simulink model "iter_imas_sc1_Zc_2"  (Simulink 8.5)
settings: Solver=ode1  StartTime=EqTime  StopTime=1e8  FixedStep=SimStep  MaxStep=5.e-3  MinStep=2e-4  RelTol=1.e-3
undefined symbols (not defined in the file): A_currterm, A_div, A_divrd, A_lim, A_vs, A_vs_hl, Acd2, B_currterm, B_div, B_divrd, B_lim, B_vs, B_vs_hl, Bcd2, C_currterm, C_div, C_divrd, C_lim, C_vs, C_vs_hl, Ccd2, D_currterm, D_div, D_divrd, D_lim, D_vs, D_vs_hl, Dcd2, Imax, key_imas, n_gaps, ncam, npf, ntur, RupRd, scr_data, SimStep, Vcspf_up, vec_imas, volt
libraries: simulink x57
(part 1 of 2)
settings Model: Creator=Kavin  ModifiedByFormat=Kavin  LastModifiedBy=Kavin  ExtModeTrigMode=oneshot  ExtModeArmWhenConnect=off  ExtModeAutoUpdateStatusClock=off
settings DataIOCC: LimitDataPoints=off  TimeSaveName=sim_time  SignalLoggingName=sigsOut
settings OptimizationCC: BooleanDataType=off  OptimizeBlockIOStorage=off  BufferReuse=off  GlobalBufferReuse=off  ExpressionFolding=off  ExpressionDepthLimit=128  LocalBlockOutputs=off  InitFltsAndDblsToZero=on
settings DebuggingCC: SaveWithParameterizedLinksMsg=none  SignalResolutionControl=TryResolveAllWithWarning  MultiTaskDSMMsg=warning  MultiTaskCondExecSysMsg=none  FcnCallInpInsideContextMsg=UseLocalSettings  StateNameClashWarn=none
settings HardwareCC: TargetUnknown=on
settings CodeAppCC: IgnoreCustomStorageClasses=off
settings GRTTargetCC: TargetFcnLib=ansi_tfl_tmw.mat

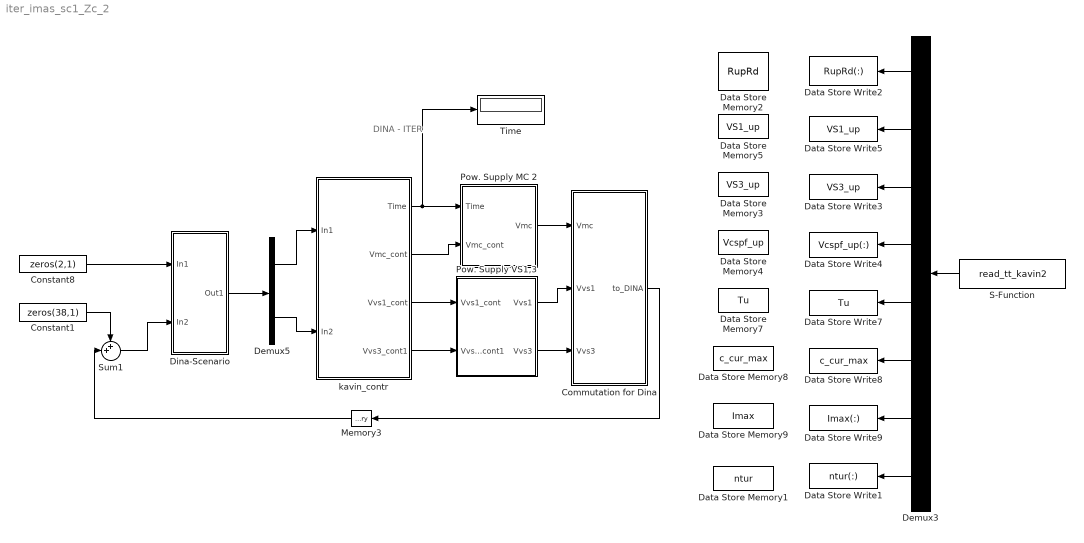
== system iter_imas_sc1_Zc_2 ==
  note: DINA - ITER
  Commutation for Dina : Subsystem
  Constant1 : Constant  Value=zeros(38,1)
  Constant8 : Constant  Value=zeros(2,1)
  Data Store Memory1 : DataStoreMemory  DataStoreName=ntur  ReadBeforeWriteMsg=warning  WriteAfterWriteMsg=warning  WriteAfterReadMsg=warning  InitialValue="[554,554,554,554,554  248.6 115.2 185.9 169.9 216.8  459.4 1]"
  Data Store Memory2 : DataStoreMemory  DataStoreName=RupRd  ReadBeforeWriteMsg=warning  WriteAfterWriteMsg=warning  WriteAfterReadMsg=warning  InitialValue=[1; ones(5,1)*1e-6]
  Data Store Memory3 : DataStoreMemory  DataStoreName=VS3_up  ReadBeforeWriteMsg=warning  WriteAfterWriteMsg=warning  WriteAfterReadMsg=warning
  Data Store Memory4 : DataStoreMemory  DataStoreName=Vcspf_up  ReadBeforeWriteMsg=warning  WriteAfterWriteMsg=warning  WriteAfterReadMsg=warning  InitialValue=zeros(11,1)
  Data Store Memory5 : DataStoreMemory  DataStoreName=VS1_up  ReadBeforeWriteMsg=warning  WriteAfterWriteMsg=warning  WriteAfterReadMsg=warning
  Data Store Memory7 : DataStoreMemory  DataStoreName=Tu  ReadBeforeWriteMsg=warning  WriteAfterWriteMsg=warning  WriteAfterReadMsg=warning
  Data Store Memory8 : DataStoreMemory  DataStoreName=c_cur_max  ReadBeforeWriteMsg=warning  WriteAfterWriteMsg=warning  WriteAfterReadMsg=warning
  Data Store Memory9 : DataStoreMemory  DataStoreName=Imax  ReadBeforeWriteMsg=warning  WriteAfterWriteMsg=warning  WriteAfterReadMsg=warning  InitialValue=ones(1,11)*1e6
  Data Store Write1 : DataStoreWrite  DataStoreName=ntur  DataStoreElements=ntur(:)
  Data Store Write2 : DataStoreWrite  DataStoreName=RupRd  DataStoreElements=RupRd(:)
  Data Store Write3 : DataStoreWrite  DataStoreName=VS3_up  DataStoreElements=VS3_up
  Data Store Write4 : DataStoreWrite  DataStoreName=Vcspf_up  DataStoreElements=Vcspf_up(:)
  Data Store Write5 : DataStoreWrite  DataStoreName=VS1_up  DataStoreElements=VS1_up
  Data Store Write7 : DataStoreWrite  DataStoreName=Tu  DataStoreElements=Tu
  Data Store Write8 : DataStoreWrite  DataStoreName=c_cur_max  DataStoreElements=c_cur_max
  Data Store Write9 : DataStoreWrite  DataStoreName=Imax  DataStoreElements=Imax(:)
  Demux3 : Demux  Outputs=[6 1 1 11 1 1 11 12]
  Demux5 : Demux  Outputs=[15 123]
  Dina-Scenario : Subsystem
  Memory3 : Memory
  Pow. Supply MC 2 : Subsystem
  Pow. Supply VS1,3 : Subsystem
  S-Function : S-Function  FunctionName=read_tt_kavin2  SFunctionModules=read_tt_kavin2_wrapper read_tt_kavin2
  Sum1 : Sum  Inputs=++|  SaturateOnIntegerOverflow=on  InputSameDT=on  OutDataTypeStr=Inherit: Same as first input
  Time : Display
  kavin_contr : Subsystem
  wires:
  Demux5/1 -> kavin_contr/1(In1)
  Demux5/2 -> kavin_contr/2(In2)
  Dina-Scenario/1(Out1) -> Demux5/1
  Constant8/1 -> Dina-Scenario/1(In1)
  Constant1/1 -> Sum1/1
  Sum1/1 -> Dina-Scenario/2(In2)
  kavin_contr/1(Time) -> Pow. Supply MC 2/1(Time), Time/1
  kavin_contr/2(Vmc_cont) -> Pow. Supply MC 2/2(Vmc_cont)
  Pow. Supply MC 2/1(Vmc) -> Commutation for Dina/1(Vmc)
  Commutation for Dina/1(to_DINA) -> Memory3/1
  S-Function/1 -> Demux3/1
  kavin_contr/3(Vvs1_cont) -> Pow. Supply VS1,3/1(Vvs1_cont)
  kavin_contr/4(Vvs3_cont1) -> Pow. Supply VS1,3/2(Vvs3_cont1)
  Pow. Supply VS1,3/2(Vvs3) -> Commutation for Dina/3(Vvs3)
  Pow. Supply VS1,3/1(Vvs1) -> Commutation for Dina/2(Vvs1)
  Demux3/8 -> Data Store Write1/1
  Demux3/7 -> Data Store Write9/1
  Demux3/6 -> Data Store Write8/1
  Demux3/5 -> Data Store Write7/1
  Demux3/4 -> Data Store Write4/1
  Demux3/3 -> Data Store Write3/1
  Demux3/2 -> Data Store Write5/1
  Demux3/1 -> Data Store Write2/1
  Memory3/1 -> Sum1/2

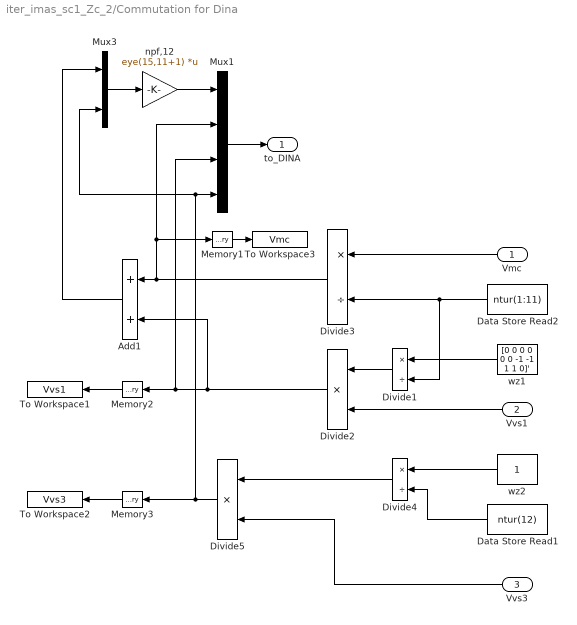
== system iter_imas_sc1_Zc_2/Commutation for Dina ==
  Vmc : Inport
  Vvs1 : Inport  Port=2
  Vvs3 : Inport  Port=3
  Add1 : Sum
  Data Store Read1 : DataStoreRead  DataStoreName=ntur  DataStoreElements=ntur(12)
  Data Store Read2 : DataStoreRead  DataStoreName=ntur  DataStoreElements=ntur(1:11)
  Divide1 : Product  Inputs=*/
  Divide2 : Product  Inputs=**
  Divide3 : Product  Inputs=*/
  Divide4 : Product  Inputs=*/
  Divide5 : Product  Inputs=**
  Memory1 : Memory
  Memory2 : Memory
  Memory3 : Memory
  Mux1 : Mux
  Mux3 : Mux  Inputs=2
  To Workspace1 : ToWorkspace  VariableName=Vvs1
  To Workspace2 : ToWorkspace  VariableName=Vvs3
  To Workspace3 : ToWorkspace  VariableName=Vmc
  npf,12 : Gain  Gain=eye(15,11+1)  Multiplication=Matrix(K*u)
  wz1 : Constant  Value=[0 0 0 0 0 0 -1 -1 1 1 0]'
  wz2 : Constant
  to_DINA : Outport
  wires:
  Divide2/1 -> Add1/2, Mux1/3, Memory2/1
  Mux1/1 -> to_DINA/1
  Add1/1 -> Mux3/1
  Mux3/1 -> npf,12/1
  npf,12/1 -> Mux1/1
  Divide3/1 -> Add1/1, Mux1/2, Memory1/1
  Vmc/1 -> Divide3/1
  Data Store Read2/1 -> Divide1/2, Divide3/2
  wz1/1 -> Divide1/1
  Divide1/1 -> Divide2/1
  Vvs1/1 -> Divide2/2
  wz2/1 -> Divide4/1
  Data Store Read1/1 -> Divide4/2
  Divide4/1 -> Divide5/1
  Vvs3/1 -> Divide5/2
  Divide5/1 -> Mux3/2, Mux1/4, Memory3/1
  Memory1/1 -> To Workspace3/1
  Memory2/1 -> To Workspace1/1
  Memory3/1 -> To Workspace2/1

== system iter_imas_sc1_Zc_2/Dina-Scenario ==
  In1 : Inport
  In2 : Inport  Port=2
  Constant15 : Constant  Value=zeros(54,1)
  Mux2 : Mux  Inputs=2
  S-Function1 : S-Function  FunctionName=dina_imas  Parameters=key_imas,vec_imas
  Terminator3 : Terminator
  To Workspace21 : ToWorkspace  VariableName=sim_shape
      settings: Decimation=DecimShape
  Out1 : Outport
  wires:
  In1/1 -> S-Function1/1
  S-Function1/2 -> Mux2/2
  S-Function1/3 -> To Workspace21/1
  S-Function1/4 -> Terminator3/1
  S-Function1/1 -> Mux2/1
  Mux2/1 -> Out1/1
  In2/1 -> S-Function1/2
  Constant15/1 -> S-Function1/3

== system iter_imas_sc1_Zc_2/Pow. Supply MC 2 ==
  Time : Inport
  Vmc_cont : Inport  Port=2
  Difference : simulink/Discrete/Difference  ICPrevInput=0.0  InputProcessing=Inherited  OutMin=[]  OutMax=[]  OutDataType=sfix(16)  OutScaling=2^-10  DoSatur=off
  Pow. Supply MC 1 : Subsystem
  Vmc : Outport
  wires:
  Time/1 -> Difference/1
  Vmc_cont/1 -> Pow. Supply MC 1/2(Vmc_cont)
  Difference/1 -> Pow. Supply MC 1/1(dt)
  Pow. Supply MC 1/1(Vmc) -> Vmc/1

== system iter_imas_sc1_Zc_2/Pow. Supply VS1,3 ==
  Vvs1_cont : Inport
  Vvs3_cont1 : Inport  Port=2
  Data Store Read1 : DataStoreRead  DataStoreName=VS1_up  DataStoreElements=VS1_up
  Data Store Read3 : DataStoreRead  DataStoreName=VS3_up  DataStoreElements=VS3_up
  Gain : Gain  Gain=-1
  Gain1 : Gain  Gain=-1
  Saturation Dynamic : simulink/Discontinuities/Saturation Dynamic  OutMin=[]  OutMax=[]  OutDataTypeStr=Inherit: Same as second input  OutDataType=fixdt(1, 16)  OutScaling=2^-10  DoSatur=off
  Saturation Dynamic1 : simulink/Discontinuities/Saturation Dynamic  OutMin=[]  OutMax=[]  OutDataTypeStr=Inherit: Same as second input  OutDataType=fixdt(1, 16)  OutScaling=2^-10  DoSatur=off
  Vvs1 : Outport
  Vvs3 : Outport  Port=2
  wires:
  Data Store Read1/1 -> Gain/1, Saturation Dynamic/1
  Gain/1 -> Saturation Dynamic/3
  Vvs1_cont/1 -> Saturation Dynamic/2
  Gain1/1 -> Saturation Dynamic1/3
  Data Store Read3/1 -> Gain1/1, Saturation Dynamic1/1
  Vvs3_cont1/1 -> Saturation Dynamic1/2
  Saturation Dynamic/1 -> Vvs1/1
  Saturation Dynamic1/1 -> Vvs3/1

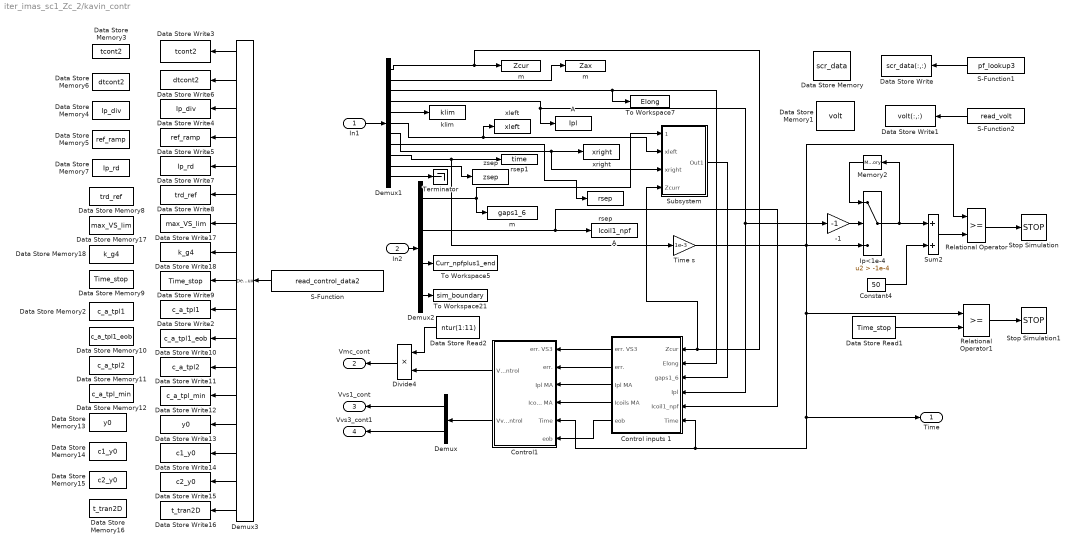
== system iter_imas_sc1_Zc_2/kavin_contr ==
  In1 : Inport
  In2 : Inport  Port=2
  -1 : Gain  Gain=-1
  A : ToWorkspace  VariableName=Ipl
  "A  " : ToWorkspace  VariableName=Icoil1_npf
  Constant4 : Constant  Value=50  VectorParams1D=off
  Control inputs 1 : Subsystem
  Control1 : Subsystem
  Data Store Memory : DataStoreMemory  DataStoreName=scr_data  ReadBeforeWriteMsg=warning  WriteAfterWriteMsg=warning  WriteAfterReadMsg=warning  InitialValue=zeros(13,500)
  Data Store Memory1 : DataStoreMemory  DataStoreName=volt  ReadBeforeWriteMsg=warning  WriteAfterWriteMsg=warning  WriteAfterReadMsg=warning  InitialValue=zeros(20,500)
  Data Store Memory10 : DataStoreMemory  DataStoreName=c_a_tpl1_eob  ReadBeforeWriteMsg=warning  WriteAfterWriteMsg=warning  WriteAfterReadMsg=warning
  Data Store Memory11 : DataStoreMemory  DataStoreName=c_a_tpl2  ReadBeforeWriteMsg=warning  WriteAfterWriteMsg=warning  WriteAfterReadMsg=warning
  Data Store Memory12 : DataStoreMemory  DataStoreName=c_a_tpl_min  ReadBeforeWriteMsg=warning  WriteAfterWriteMsg=warning  WriteAfterReadMsg=warning
  Data Store Memory13 : DataStoreMemory  DataStoreName=y0  ReadBeforeWriteMsg=warning  WriteAfterWriteMsg=warning  WriteAfterReadMsg=warning
  Data Store Memory14 : DataStoreMemory  DataStoreName=c1_y0  ReadBeforeWriteMsg=warning  WriteAfterWriteMsg=warning  WriteAfterReadMsg=warning
  Data Store Memory15 : DataStoreMemory  DataStoreName=c2_y0  ReadBeforeWriteMsg=warning  WriteAfterWriteMsg=warning  WriteAfterReadMsg=warning
  Data Store Memory16 : DataStoreMemory  DataStoreName=t_tran2D  ReadBeforeWriteMsg=warning  WriteAfterWriteMsg=warning  WriteAfterReadMsg=warning
  Data Store Memory17 : DataStoreMemory  DataStoreName=max_VS_lim  ReadBeforeWriteMsg=warning  WriteAfterWriteMsg=warning  WriteAfterReadMsg=warning
  Data Store Memory18 : DataStoreMemory  DataStoreName=k_g4  ReadBeforeWriteMsg=warning  WriteAfterWriteMsg=warning  WriteAfterReadMsg=warning
  Data Store Memory2 : DataStoreMemory  DataStoreName=c_a_tpl1  ReadBeforeWriteMsg=warning  WriteAfterWriteMsg=warning  WriteAfterReadMsg=warning
  Data Store Memory3 : DataStoreMemory  DataStoreName=tcont2  ReadBeforeWriteMsg=warning  WriteAfterWriteMsg=warning  WriteAfterReadMsg=warning
  Data Store Memory4 : DataStoreMemory  DataStoreName=Ip_div  ReadBeforeWriteMsg=warning  WriteAfterWriteMsg=warning  WriteAfterReadMsg=warning  InitialValue=0.1
  Data Store Memory5 : DataStoreMemory  DataStoreName=ref_ramp  ReadBeforeWriteMsg=warning  WriteAfterWriteMsg=warning  WriteAfterReadMsg=warning  InitialValue=1e-3
  Data Store Memory6 : DataStoreMemory  DataStoreName=dtcont2  ReadBeforeWriteMsg=warning  WriteAfterWriteMsg=warning  WriteAfterReadMsg=warning  InitialValue=1e-3
  Data Store Memory7 : DataStoreMemory  DataStoreName=Ip_rd  ReadBeforeWriteMsg=warning  WriteAfterWriteMsg=warning  WriteAfterReadMsg=warning
  Data Store Memory8 : DataStoreMemory  DataStoreName=trd_ref  ReadBeforeWriteMsg=warning  WriteAfterWriteMsg=warning  WriteAfterReadMsg=warning
  Data Store Memory9 : DataStoreMemory  DataStoreName=Time_stop  ReadBeforeWriteMsg=warning  WriteAfterWriteMsg=warning  WriteAfterReadMsg=warning
  Data Store Read1 : DataStoreRead  DataStoreName=Time_stop  DataStoreElements=Time_stop
  Data Store Read2 : DataStoreRead  DataStoreName=ntur  DataStoreElements=ntur(1:11)
  Data Store Write : DataStoreWrite  DataStoreName=scr_data  DataStoreElements=scr_data(:,:)
  Data Store Write1 : DataStoreWrite  DataStoreName=volt  DataStoreElements=volt(:,:)
  Data Store Write10 : DataStoreWrite  DataStoreName=c_a_tpl1_eob  DataStoreElements=c_a_tpl1_eob
  Data Store Write11 : DataStoreWrite  DataStoreName=c_a_tpl2  DataStoreElements=c_a_tpl2
  Data Store Write12 : DataStoreWrite  DataStoreName=c_a_tpl_min  DataStoreElements=c_a_tpl_min
  Data Store Write13 : DataStoreWrite  DataStoreName=y0  DataStoreElements=y0
  Data Store Write14 : DataStoreWrite  DataStoreName=c1_y0  DataStoreElements=c1_y0
  Data Store Write15 : DataStoreWrite  DataStoreName=c2_y0  DataStoreElements=c2_y0
  Data Store Write16 : DataStoreWrite  DataStoreName=t_tran2D  DataStoreElements=t_tran2D
  Data Store Write17 : DataStoreWrite  DataStoreName=max_VS_lim  DataStoreElements=max_VS_lim
  Data Store Write18 : DataStoreWrite  DataStoreName=k_g4  DataStoreElements=k_g4
  Data Store Write2 : DataStoreWrite  DataStoreName=c_a_tpl1  DataStoreElements=c_a_tpl1
  Data Store Write3 : DataStoreWrite  DataStoreName=tcont2  DataStoreElements=tcont2
  Data Store Write4 : DataStoreWrite  DataStoreName=Ip_div  DataStoreElements=Ip_div
  Data Store Write5 : DataStoreWrite  DataStoreName=ref_ramp  DataStoreElements=ref_ramp
  Data Store Write6 : DataStoreWrite  DataStoreName=dtcont2  DataStoreElements=dtcont2
  Data Store Write7 : DataStoreWrite  DataStoreName=Ip_rd  DataStoreElements=Ip_rd
  Data Store Write8 : DataStoreWrite  DataStoreName=trd_ref  DataStoreElements=trd_ref
  Data Store Write9 : DataStoreWrite  DataStoreName=Time_stop  DataStoreElements=Time_stop
  Demux : Demux  Outputs=2
  Demux1 : Demux  Outputs=[1 1 1 1 1 1 1 1 1 1 5 ]
  Demux2 : Demux  Outputs=[n_gaps npf ncam 2]
  Demux3 : Demux  Outputs=ones(1,17)
  Divide4 : Product  Inputs=**
  "Ip<1e-4 " : Switch  Criteria=u2 > Threshold  Threshold=-1e-4
  Memory2 : Memory
  Relational Operator : RelationalOperator  OutDataTypeStr=boolean
  Relational Operator1 : RelationalOperator  OutDataTypeStr=boolean
  S-Function : S-Function  FunctionName=read_control_data2  SFunctionModules=read_control_data2_wrapper read_control_data2
  S-Function1 : S-Function  FunctionName=pf_lookup3  Parameters=1  SFunctionModules='pf_lookup3_wrapper read_pf'
  S-Function2 : S-Function  FunctionName=read_volt  Parameters=12  SFunctionModules='read_volt_wrapper read_volt'
  Stop Simulation : Stop
  Stop Simulation1 : Stop
  Subsystem : Subsystem
  Sum2 : Sum
  Terminator : Terminator
  Time s : Gain  Gain=1e-3
  To Workspace21 : ToWorkspace  VariableName=sim_boundary
      settings: Decimation=DecimShape
  To Workspace5 : ToWorkspace  VariableName=Curr_npfplus1_end
  To Workspace7 : ToWorkspace  VariableName=Elong
  klim : ToWorkspace  VariableName=klim
  m : ToWorkspace  VariableName=gaps1_6
  "m  " : ToWorkspace  VariableName=Zax
  "m   " : ToWorkspace  VariableName=Zcur
  rsep : ToWorkspace  VariableName=rsep
  rsep1 : ToWorkspace  VariableName=time
  xleft : ToWorkspace  VariableName=xleft
  xright : ToWorkspace  VariableName=xright
  zsep : ToWorkspace  VariableName=zsep
  Time : Outport
  Vmc_cont : Outport  Port=2
  Vvs1_cont : Outport  Port=3
  Vvs3_cont1 : Outport  Port=4
  wires:
  Demux1/2 -> "m  "/1
  Demux1/1 -> Subsystem/4(Zcurr), Control inputs 1/1(Zcur), "m   "/1
  Demux1/3 -> To Workspace7/1, Control inputs 1/2(Elong)
  Demux2/4 -> To Workspace21/1
  Demux1/4 -> A/1, Control inputs 1/4(Ipl), -1/1
  Demux2/3 -> To Workspace5/1
  Demux2/2 -> "A  "/1, Control inputs 1/5(Icoil1_npf)
  Control inputs 1/2(err.) -> Control1/2(err.)
  Control inputs 1/4(Icoils MA) -> Control1/4(Icoils MA)
  In1/1 -> Demux1/1
  In2/1 -> Demux2/1
  Demux1/5 -> klim/1
  Demux1/6 -> Subsystem/2(xleft), xleft/1
  Demux1/7 -> Subsystem/3(xright), xright/1
  Demux1/8 -> rsep/1
  Demux2/1 -> Subsystem/1(gaps1_6), m/1
  Subsystem/1(Out1) -> Control inputs 1/3(gaps1_6)
  Demux1/11 -> Terminator/1
  Demux1/9 -> rsep1/1, Time s/1
  Demux1/10 -> zsep/1
  Time s/1 -> "Ip<1e-4 "/3, Relational Operator/1, Control1/5(Time), Control inputs 1/6(Time), Time/1, Relational Operator1/1
  Relational Operator/1 -> Stop Simulation/1
  -1/1 -> "Ip<1e-4 "/2
  "Ip<1e-4 "/1 -> Memory2/1, Sum2/1
  Memory2/1 -> "Ip<1e-4 "/1
  Sum2/1 -> Relational Operator/2
  Relational Operator1/1 -> Stop Simulation1/1
  Data Store Read1/1 -> Relational Operator1/2
  Control1/2(Vvs control) -> Demux/1
  S-Function1/1 -> Data Store Write/1
  S-Function2/1 -> Data Store Write1/1
  Demux/1 -> Vvs1_cont/1
  Demux/2 -> Vvs3_cont1/1
  Divide4/1 -> Vmc_cont/1
  Control1/1(Vmc control) -> Divide4/2
  Data Store Read2/1 -> Divide4/1
  Control inputs 1/1(err. VS3) -> Control1/1(err. VS3)
  Control inputs 1/3(Ipl MA) -> Control1/3(Ipl MA)
  Control inputs 1/5(eob) -> Control1/6(eob)
  S-Function/1 -> Demux3/1
  Demux3/6 -> Data Store Write8/1
  Demux3/5 -> Data Store Write7/1
  Demux3/4 -> Data Store Write5/1
  Demux3/3 -> Data Store Write4/1
  Demux3/2 -> Data Store Write6/1
  Demux3/1 -> Data Store Write3/1
  Demux3/9 -> Data Store Write9/1
  Demux3/10 -> Data Store Write2/1
  Demux3/11 -> Data Store Write10/1
  Demux3/12 -> Data Store Write11/1
  Demux3/13 -> Data Store Write12/1
  Demux3/14 -> Data Store Write13/1
  Demux3/15 -> Data Store Write14/1
  Demux3/16 -> Data Store Write15/1
  Demux3/17 -> Data Store Write16/1
  Demux3/7 -> Data Store Write17/1
  Demux3/8 -> Data Store Write18/1
  Constant4/1 -> Sum2/2

== system iter_imas_sc1_Zc_2/Pow. Supply MC 2/Pow. Supply MC 1 ==
  dt : Inport
  Vmc_cont : Inport  Port=2
  Add1 : Sum  Inputs=-+
  Add2 : Sum
  Divide : Product  Inputs=*/
  Divide1 : Product  Inputs=**
  MC rate : Subsystem
  MC satur. : Subsystem
  Memory1 : Memory
  Vmc : Outport
  wires:
  dt/1 -> Divide/2, Divide1/2
  Add1/1 -> Divide/1
  Vmc_cont/1 -> Add1/2
  Divide1/1 -> Add2/2
  Memory1/1 -> Add2/1, Add1/1
  MC satur./1(Out1) -> Memory1/1, Vmc/1
  Add2/1 -> MC satur./1(In1)
  Divide/1 -> MC rate/1(In1)
  MC rate/1(Out1) -> Divide1/1

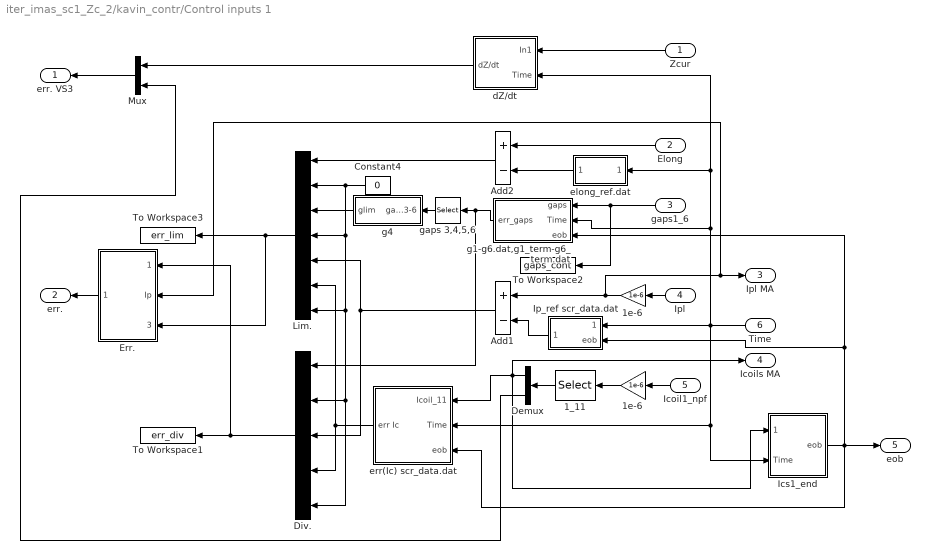
== system iter_imas_sc1_Zc_2/kavin_contr/Control inputs 1 ==
  Zcur : Inport
  Elong : Inport  Port=2
  gaps1_6 : Inport  Port=3
  Ipl : Inport  Port=4
  Icoil1_npf : Inport  Port=5
  Time : Inport  Port=6
  1_11 : Selector  InputPortWidth=15  Indices=[1:11+1]
  1e-6 : Gain  Gain=1e-6
  "1e-6   " : Gain  Gain=1e-6
  Add1 : Sum  Inputs=+-
  Add2 : Sum  Inputs=+-
  Constant4 : Constant  Value=0  VectorParams1D=off
  Demux : Demux  Outputs=[11 1]
  "Div. " : Mux  Inputs=5
  Err. : Subsystem
  Ics1_end : Subsystem
  Ip_ref scr_data.dat : Subsystem
  "Lim. " : Mux  Inputs=7
  Mux : Mux  Inputs=2
  To Workspace1 : ToWorkspace  VariableName=err_div
  To Workspace2 : ToWorkspace  VariableName=gaps_cont
  To Workspace3 : ToWorkspace  VariableName=err_lim
  dZ/dt : Subsystem
  elong_ref.dat : Subsystem
  err(Ic) scr_data.dat : Subsystem
  g1-g6.dat,g1_term-g6_term.dat : Subsystem
  g4 : Subsystem
  gaps 3,4,5,6 : Selector  InputPortWidth=6  Indices=[3:6]
  err. VS3 : Outport
  err. : Outport  Port=2
  Ipl MA : Outport  Port=3
  Icoils MA : Outport  Port=4
  eob : Outport  Port=5
  wires:
  Zcur/1 -> dZ/dt/1(In1)
  gaps1_6/1 -> To Workspace2/1, g1-g6.dat,g1_term-g6_term.dat/1(gaps)
  Ipl/1 -> 1e-6/1
  Icoil1_npf/1 -> "1e-6   "/1
  "1e-6   "/1 -> 1_11/1
  1_11/1 -> Demux/1
  Elong/1 -> Add2/1
  Ip_ref scr_data.dat/1(Ip ref) -> Add1/2
  1e-6/1 -> Add1/1, Err./2(Ip), Ipl MA/1
  Demux/1 -> Ics1_end/1(Icoils,MA), Icoils MA/1, err(Ic) scr_data.dat/1(Icoil_11)
  Add2/1 -> "Lim. "/1
  Constant4/1 -> "Lim. "/2, "Lim. "/4, "Lim. "/7, "Div. "/2, "Div. "/5
  Add1/1 -> "Lim. "/5, "Div. "/3
  err(Ic) scr_data.dat/1(err Ic) -> "Div. "/4, "Lim. "/6
  g1-g6.dat,g1_term-g6_term.dat/1(err_gaps) -> gaps 3,4,5,6/1, "Div. "/1
  Demux/2 -> Mux/2
  Mux/1 -> err. VS3/1
  "Div. "/1 -> Err./1(err. div.), To Workspace1/1
  "Lim. "/1 -> Err./3(err. lim.), To Workspace3/1
  Err./1(errors) -> err./1
  elong_ref.dat/1(Elong) -> Add2/2
  dZ/dt/1(dZ/dt) -> Mux/1
  Time/1 -> elong_ref.dat/1(Time), dZ/dt/2(Time), g1-g6.dat,g1_term-g6_term.dat/2(Time), err(Ic) scr_data.dat/2(Time), Ics1_end/2(Time), Ip_ref scr_data.dat/1(Time)
  Ics1_end/1(eob) -> err(Ic) scr_data.dat/3(eob), g1-g6.dat,g1_term-g6_term.dat/3(eob), Ip_ref scr_data.dat/2(eob), eob/1
  gaps 3,4,5,6/1 -> g4/1(gaps3-6)
  g4/1(glim) -> "Lim. "/3

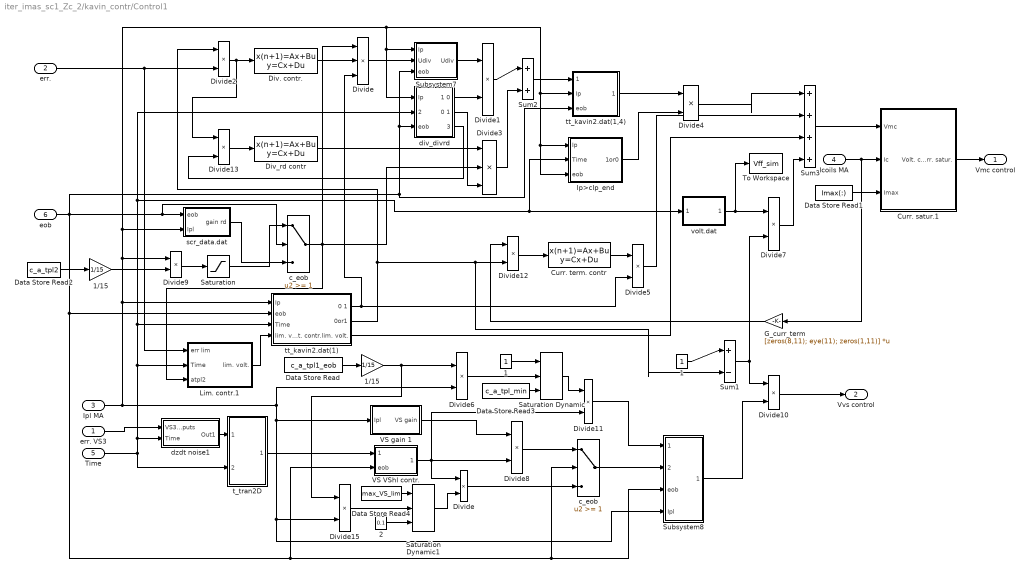
== system iter_imas_sc1_Zc_2/kavin_contr/Control1 ==
  err. VS3 : Inport
  err. : Inport  Port=2
  Ipl MA : Inport  Port=3
  Icoils MA : Inport  Port=4
  Time : Inport  Port=5
  eob : Inport  Port=6
  " 1/15" : Gain  Gain=1/15
  " 1/15 " : Gain  Gain=1/15
  " tt_kavin2.dat(1)" : Subsystem
  1 : Constant
  "1 " : Constant
  2 : Constant  Value=0.1
  Curr. satur.1 : Subsystem
  Curr. term. contr : DiscreteStateSpace  A=A_currterm  B=B_currterm  C=C_currterm  D=D_currterm  SampleTime=SimStep
  Data Store Read : DataStoreRead  DataStoreName=c_a_tpl1_eob  DataStoreElements=c_a_tpl1_eob
  Data Store Read1 : DataStoreRead  DataStoreName=Imax  DataStoreElements=Imax(:)
  Data Store Read2 : DataStoreRead  DataStoreName=c_a_tpl2  DataStoreElements=c_a_tpl2
  Data Store Read3 : DataStoreRead  DataStoreName=c_a_tpl_min  DataStoreElements=c_a_tpl_min
  Data Store Read4 : DataStoreRead  DataStoreName=max_VS_lim  DataStoreElements=max_VS_lim
  Div. contr. : DiscreteStateSpace  A=A_div  B=B_div  C=C_div  D=D_div  SampleTime=SimStep
  Div_rd contr : DiscreteStateSpace  A=A_divrd  B=B_divrd  C=C_divrd  D=D_divrd  SampleTime=SimStep
  Divide : Product  Inputs=***
  "Divide " : Product  Inputs=**
  Divide{1..2,4..13,15} (13 alike) : Product  Inputs=**
  Divide3 : Product  Inputs=***
  G_curr_term : Gain  Gain=[zeros(8,11); eye(11); zeros(1,11)]  Multiplication=Matrix(K*u)
  Ip>cIp_end : Subsystem
  Lim. contr.1 : Subsystem
  Saturation : Saturate  UpperLimit=1  LowerLimit=0
  Saturation Dynamic : simulink/Discontinuities/Saturation Dynamic  OutMin=[]  OutMax=[]  OutDataTypeStr=Inherit: Same as second input  OutDataType=fixdt(1, 16)  OutScaling=2^-10  DoSatur=off
  Saturation Dynamic1 : simulink/Discontinuities/Saturation Dynamic  OutMin=[]  OutMax=[]  OutDataTypeStr=Inherit: Same as second input  OutDataType=fixdt(1, 16)  OutScaling=2^-10  DoSatur=off
  Subsystem7 : Subsystem
  Subsystem8 : Subsystem
  Sum1 : Sum  Inputs=|+-
  Sum2 : Sum  Inputs=|++
  Sum3 : Sum  Inputs=|++++
  To Workspace : ToWorkspace  VariableName=Vff_sim  SampleTime=-1
  VS VShl contr. : Subsystem
  VS gain 1 : Subsystem
  c_eob : Switch  Threshold=1
  "c_eob " : Switch  Threshold=1
  div_divrd : Subsystem
  dzdt noise1 : Subsystem
  scr_data.dat : Subsystem
  t_tran2D : Subsystem
  tt_kavin2.dat(1,4) : Subsystem
  volt.dat : Subsystem
  Vmc control : Outport
  Vvs control : Outport  Port=2
  wires:
  err./1 -> Lim. contr.1/1(err lim), Divide2/2
  Div. contr./1 -> Divide/2
  Divide/1 -> Subsystem7/2(Udiv)
  Divide13/1 -> Div_rd contr/1
  c_eob/1 -> Divide/1, Divide3/2, Lim. contr.1/3(atpl2)
  Div_rd contr/1 -> Divide3/1
  Divide1/1 -> Sum2/1
  Divide3/1 -> Sum2/2
  Divide4/1 -> Sum3/1
  Curr. term. contr/1 -> Divide5/1
  Divide5/1 -> Sum3/2
  volt.dat/1(ref. volt.) -> Divide7/1, To Workspace/1
  Divide7/1 -> Sum3/4
  Divide10/1 -> Vvs control/1
  Icoils MA/1 -> Curr. satur.1/2(Ic), G_curr_term/1
  VS VShl contr./1(Out1) -> Divide8/2, "Divide "/1, Divide11/2
  VS gain 1/1(VS gain) -> Divide8/1
  "c_eob "/1 -> Subsystem8/2(VSeob)
  Divide11/1 -> Subsystem8/1(VSrd)
  err. VS3/1 -> dzdt noise1/1(VS3 inputs)
  Subsystem8/1(Out1) -> Divide10/2
  Subsystem7/1("Udiv ") -> Divide1/1
  Divide2/1 -> Divide13/1, Div. contr./1
  Divide12/1 -> Curr. term. contr/1
  Time/1 -> t_tran2D/2(Time), div_divrd/2(Time), volt.dat/1(Time), Ip>cIp_end/2(Time), " tt_kavin2.dat(1)"/3(Time), Lim. contr.1/2(Time), dzdt noise1/2(Time)
  div_divrd/1(1 0) -> Divide1/2
  div_divrd/2(0 1) -> Divide3/3
  div_divrd/3(0or1) -> Divide13/2
  Ip>cIp_end/1(1or0) -> Divide4/2
  eob/1 -> tt_kavin2.dat(1,4)/3(eob), Subsystem7/3(eob), div_divrd/3(eob), " tt_kavin2.dat(1)"/2(eob), Subsystem8/3(eob), "c_eob "/2, VS VShl contr./2(eob), scr_data.dat/1(eob), c_eob/2
  scr_data.dat/1(gain rd) -> c_eob/3
  Saturation/1 -> c_eob/1
  Divide8/1 -> "c_eob "/1
  "Divide "/1 -> "c_eob "/3
  Sum2/1 -> tt_kavin2.dat(1,4)/1(Vdivrd)
  tt_kavin2.dat(1,4)/1("Vdivrd ") -> Divide4/1
  dzdt noise1/1(Out1) -> t_tran2D/1(Noise,VS3)
  t_tran2D/1(Out1) -> VS VShl contr./1(err VS)
  Data Store Read/1 -> " 1/15"/1
  " 1/15"/1 -> Divide15/1, Divide6/1
  Data Store Read2/1 -> " 1/15 "/1
  Divide9/1 -> Saturation/1
  " 1/15 "/1 -> Divide9/2
  Divide6/1 -> Saturation Dynamic/2
  Saturation Dynamic/1 -> Divide11/1
  Data Store Read3/1 -> Saturation Dynamic/3
  1/1 -> Saturation Dynamic/1
  Saturation Dynamic1/1 -> "Divide "/2
  Lim. contr.1/1(lim. volt.) -> " tt_kavin2.dat(1)"/4(lim. volt. contr.)
  " tt_kavin2.dat(1)"/1(0 1) -> Divide/3, Divide5/2
  " tt_kavin2.dat(1)"/2(0or1) -> Sum1/2, Divide12/2, Divide2/1
  G_curr_term/1 -> Divide12/1
  "1 "/1 -> Sum1/1
  Sum1/1 -> Divide10/1, Divide7/2
  Divide15/1 -> Saturation Dynamic1/2
  Ipl MA/1 -> Divide9/1, scr_data.dat/2(Ipl), Ip>cIp_end/3(eob), Ip>cIp_end/1(Ip), tt_kavin2.dat(1,4)/2(Ip), div_divrd/1(Ip), Subsystem7/1(Ip), " tt_kavin2.dat(1)"/1(Ip), Subsystem8/4(Ipl), Divide15/2, VS gain 1/1(Ipl), Divide6/2
  Curr. satur.1/1(Volt. curr. satur.) -> Vmc control/1
  Sum3/1 -> Curr. satur.1/1(Vmc)
  Data Store Read1/1 -> Curr. satur.1/3(Imax)
  Data Store Read4/1 -> Saturation Dynamic1/1
  2/1 -> Saturation Dynamic1/3
  " tt_kavin2.dat(1)"/3("lim. volt. ") -> Sum3/3

== system iter_imas_sc1_Zc_2/kavin_contr/Subsystem ==
  gaps1_6 : Inport
  xleft : Inport  Port=2
  xright : Inport  Port=3
  Zcurr : Inport  Port=4
  Mux3 : Mux
  Selector : Selector  InputPortWidth=9  Indices=[1 2 7 4 9 8]
  Out1 : Outport
  wires:
  gaps1_6/1 -> Mux3/1
  xright/1 -> Mux3/2
  Mux3/1 -> Selector/1
  Selector/1 -> Out1/1
  xleft/1 -> Mux3/3
  Zcurr/1 -> Mux3/4

== system iter_imas_sc1_Zc_2/Pow. Supply MC 2/Pow. Supply MC 1/MC rate ==
  In1 : Inport
  -1 : Gain  Gain=-1
  2 : Gain  Gain=2
  Data Store Read1 : DataStoreRead  DataStoreName=Vcspf_up  DataStoreElements=Vcspf_up(:)
  Data Store Read3 : DataStoreRead  DataStoreName=Tu  DataStoreElements=Tu
  Divide1 : Product  Inputs=*/
  Saturation Dynamic : simulink/Discontinuities/Saturation Dynamic  OutMin=[]  OutMax=[]  OutDataTypeStr=Inherit: Same as second input  OutDataType=fixdt(1, 16)  OutScaling=2^-10  DoSatur=off
  Out1 : Outport
  wires:
  Saturation Dynamic/1 -> Out1/1
  In1/1 -> Saturation Dynamic/2
  Divide1/1 -> Saturation Dynamic/1, -1/1
  Data Store Read1/1 -> 2/1
  2/1 -> Divide1/1
  Data Store Read3/1 -> Divide1/2
  -1/1 -> Saturation Dynamic/3

== system iter_imas_sc1_Zc_2/Pow. Supply MC 2/Pow. Supply MC 1/MC satur. ==
  In1 : Inport
  Data Store Read1 : DataStoreRead  DataStoreName=Vcspf_up  DataStoreElements=Vcspf_up(:)
  Gain : Gain  Gain=-1
  Saturation Dynamic : simulink/Discontinuities/Saturation Dynamic  OutMin=[]  OutMax=[]  OutDataTypeStr=Inherit: Same as second input  OutDataType=fixdt(1, 16)  OutScaling=2^-10  DoSatur=off
  Out1 : Outport
  wires:
  Data Store Read1/1 -> Gain/1, Saturation Dynamic/1
  Gain/1 -> Saturation Dynamic/3
  In1/1 -> Saturation Dynamic/2
  Saturation Dynamic/1 -> Out1/1

== system iter_imas_sc1_Zc_2/kavin_contr/Control inputs 1/Err. ==
  err. div. : Inport
  Ip : Inport  Port=2
  err. lim. : Inport  Port=3
  1 : Switch  Threshold=1
  Data Store Read1 : DataStoreRead  DataStoreName=Ip_div  DataStoreElements=Ip_div
  Relational Operator : RelationalOperator  Operator=>  OutDataTypeStr=float('double')
  Trigger : Subsystem
  errors : Outport
  wires:
  err. lim./1 -> 1/3
  1/1 -> errors/1
  err. div./1 -> 1/1
  Relational Operator/1 -> Trigger/1(Input)
  Trigger/1(State) -> 1/2
  Ip/1 -> Relational Operator/1
  Data Store Read1/1 -> Relational Operator/2

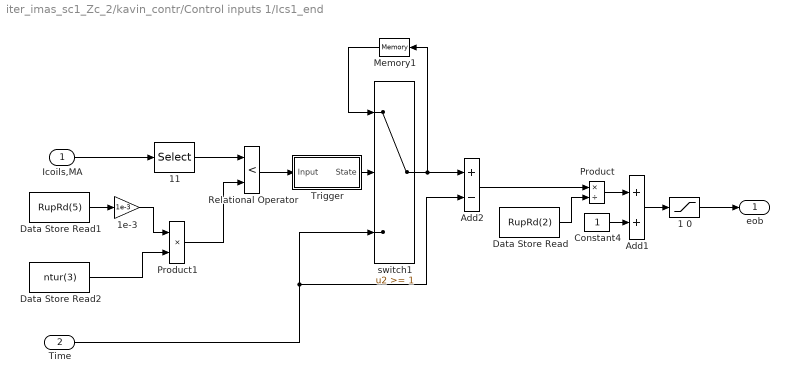
== system iter_imas_sc1_Zc_2/kavin_contr/Control inputs 1/Ics1_end ==
  Icoils,MA : Inport
  Time : Inport  Port=2
  1 0 : Saturate  UpperLimit=1  LowerLimit=0
  11 : Selector  InputPortWidth=11  Indices=3
  1e-3 : Gain  Gain=1e-3
  Add1 : Sum
  Add2 : Sum  Inputs=+-
  Constant4 : Constant  VectorParams1D=off
  Data Store Read : DataStoreRead  DataStoreName=RupRd  DataStoreElements=RupRd(2)
  Data Store Read1 : DataStoreRead  DataStoreName=RupRd  DataStoreElements=RupRd(5)
  Data Store Read2 : DataStoreRead  DataStoreName=ntur  DataStoreElements=ntur(3)
  Memory1 : Memory
  Product : Product  Inputs=*/
  Product1 : Product  Inputs=**
  Relational Operator : RelationalOperator  Operator=<  OutDataTypeStr=float('double')
  Trigger : Subsystem
  switch1 : Switch  Threshold=1
  eob : Outport
  wires:
  1 0/1 -> eob/1
  11/1 -> Relational Operator/1
  Icoils,MA/1 -> 11/1
  Data Store Read1/1 -> 1e-3/1
  1e-3/1 -> Product1/1
  Data Store Read2/1 -> Product1/2
  Product1/1 -> Relational Operator/2
  Time/1 -> Add2/2, switch1/3
  switch1/1 -> Memory1/1, Add2/1
  Add2/1 -> Product/1
  Product/1 -> Add1/1
  Constant4/1 -> Add1/2
  Add1/1 -> 1 0/1
  Data Store Read/1 -> Product/2
  Trigger/1(State) -> switch1/2
  Relational Operator/1 -> Trigger/1(Input)
  Memory1/1 -> switch1/1

== system iter_imas_sc1_Zc_2/kavin_contr/Control inputs 1/Ip_ref scr_data.dat ==
  Time : Inport
  eob : Inport  Port=2
  Data Store Read : DataStoreRead  DataStoreName=scr_data  DataStoreElements=scr_data(1,:)
  Data Store Read1 : DataStoreRead  DataStoreName=scr_data  DataStoreElements=scr_data(2,:)
  Divide6 : Product  Inputs=**
  Ipref : simulink/Lookup Tables/Lookup Table Dynamic  LookUpMeth=Interpolation-Use End Values  OutDataTypeStr=fixdt('double')  OutputDataTypeScalingMode=Specify via dialog  OutDataType=fixdt('double')  OutScaling=2^-10  DoSatur=off
  Memory1 : Memory
  c_eob : Switch  Threshold=1
  Ip ref : Outport
  wires:
  c_eob/1 -> Divide6/1, Memory1/1
  Divide6/1 -> Ip ref/1
  eob/1 -> c_eob/2, Divide6/2
  Memory1/1 -> c_eob/3
  Data Store Read1/1 -> Ipref/3
  Data Store Read/1 -> Ipref/2
  Ipref/1 -> c_eob/1
  Time/1 -> Ipref/1

== system iter_imas_sc1_Zc_2/kavin_contr/Control inputs 1/dZ/dt ==
  In1 : Inport
  Time : Inport  Port=2
  Difference : simulink/Discrete/Difference  ICPrevInput=0.0  InputProcessing=Inherited  OutMin=[]  OutMax=[]  OutDataType=sfix(16)  OutScaling=2^-10  DoSatur=off
  Difference1 : simulink/Discrete/Difference  ICPrevInput=0  InputProcessing=Inherited  OutMin=[]  OutMax=[]  OutDataType=sfix(16)  OutScaling=2^-10  DoSatur=off
  Divide : Product  Inputs=*/
  dZ/dt : Outport
  wires:
  In1/1 -> Difference/1
  Time/1 -> Difference1/1
  Difference/1 -> Divide/1
  Difference1/1 -> Divide/2
  Divide/1 -> dZ/dt/1

== system iter_imas_sc1_Zc_2/kavin_contr/Control inputs 1/elong_ref.dat ==
  Time : Inport
  S-Function1 : S-Function  FunctionName=read_gaps  Parameters=0  SFunctionModules='read_gaps_wrapper read_gaps'
  Selector : Selector  NumberOfDimensions=2  InputPortWidth=13  IndexOptions=Index vector (dialog),Select all  Indices=2,1  OutputSizes=1,1
  Selector1 : Selector  NumberOfDimensions=2  InputPortWidth=13  IndexOptions=Index vector (dialog),Select all  Indices=1,1  OutputSizes=1,1
  elong : simulink/Lookup Tables/Lookup Table Dynamic  LookUpMeth=Interpolation-Use End Values  OutDataTypeStr=fixdt('double')  OutputDataTypeScalingMode=Specify via dialog  OutDataType=fixdt('double')  OutScaling=2^-10  DoSatur=off
  Elong : Outport
  wires:
  elong/1 -> Elong/1
  Selector/1 -> elong/3
  Selector1/1 -> elong/2
  Time/1 -> elong/1
  S-Function1/1 -> Selector/1, Selector1/1

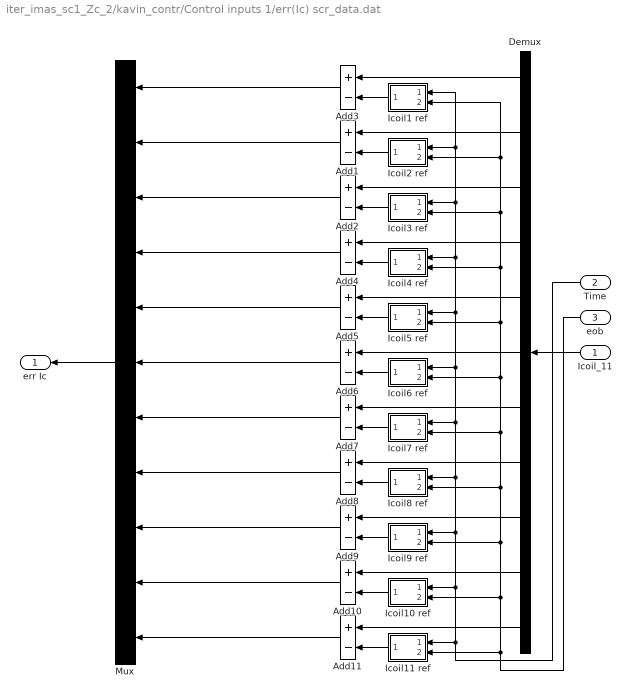
== system iter_imas_sc1_Zc_2/kavin_contr/Control inputs 1/err(Ic) scr_data.dat ==
  Icoil_11 : Inport
  Time : Inport  Port=2
  eob : Inport  Port=3
  Add{1..11} (11 alike) : Sum  Inputs=+-
  Demux : Demux  Outputs=11
  Icoil1 ref : Subsystem
  Icoil10 ref : Subsystem
  Icoil11 ref : Subsystem
  Icoil2 ref : Subsystem
  Icoil3 ref : Subsystem
  Icoil4 ref : Subsystem
  Icoil5 ref : Subsystem
  Icoil6 ref : Subsystem
  Icoil7 ref : Subsystem
  Icoil8 ref : Subsystem
  Icoil9 ref : Subsystem
  Mux : Mux  Inputs=11
  err Ic : Outport
  wires:
  Icoil_11/1 -> Demux/1
  Demux/1 -> Add3/1
  Icoil2 ref/1(Out) -> Add1/2
  Demux/2 -> Add1/1
  Demux/3 -> Add2/1
  Icoil3 ref/1(Out) -> Add2/2
  Icoil4 ref/1(Out) -> Add4/2
  Demux/4 -> Add4/1
  Icoil5 ref/1(Out) -> Add5/2
  Demux/5 -> Add5/1
  Icoil6 ref/1(Out) -> Add6/2
  Demux/6 -> Add6/1
  Icoil7 ref/1(Out) -> Add7/2
  Demux/7 -> Add7/1
  Icoil8 ref/1(Out) -> Add8/2
  Demux/8 -> Add8/1
  Icoil9 ref/1(Out) -> Add9/2
  Demux/9 -> Add9/1
  Icoil10 ref/1(Out1) -> Add10/2
  Demux/10 -> Add10/1
  Icoil11 ref/1(Out) -> Add11/2
  Demux/11 -> Add11/1
  Add3/1 -> Mux/1
  Add1/1 -> Mux/2
  Add2/1 -> Mux/3
  Add4/1 -> Mux/4
  Add6/1 -> Mux/6
  Add7/1 -> Mux/7
  Add8/1 -> Mux/8
  Add9/1 -> Mux/9
  Add10/1 -> Mux/10
  Add11/1 -> Mux/11
  Mux/1 -> err Ic/1
  Add5/1 -> Mux/5
  Icoil1 ref/1(Out) -> Add3/2
  eob/1 -> Icoil11 ref/2(eob), Icoil10 ref/2(eob), Icoil9 ref/2(eob), Icoil8 ref/2(eob), Icoil7 ref/2(eob), Icoil6 ref/2(eob), Icoil5 ref/2(eob), Icoil4 ref/2(eob), Icoil3 ref/2(eob), Icoil2 ref/2(eob), Icoil1 ref/2(eob)
  Time/1 -> Icoil11 ref/1(Time), Icoil10 ref/1(Time), Icoil9 ref/1(Time), Icoil8 ref/1(Time), Icoil7 ref/1(Time), Icoil6 ref/1(Time), Icoil5 ref/1(Time), Icoil4 ref/1(Time), Icoil3 ref/1(Time), Icoil2 ref/1(Time), Icoil1 ref/1(Time)

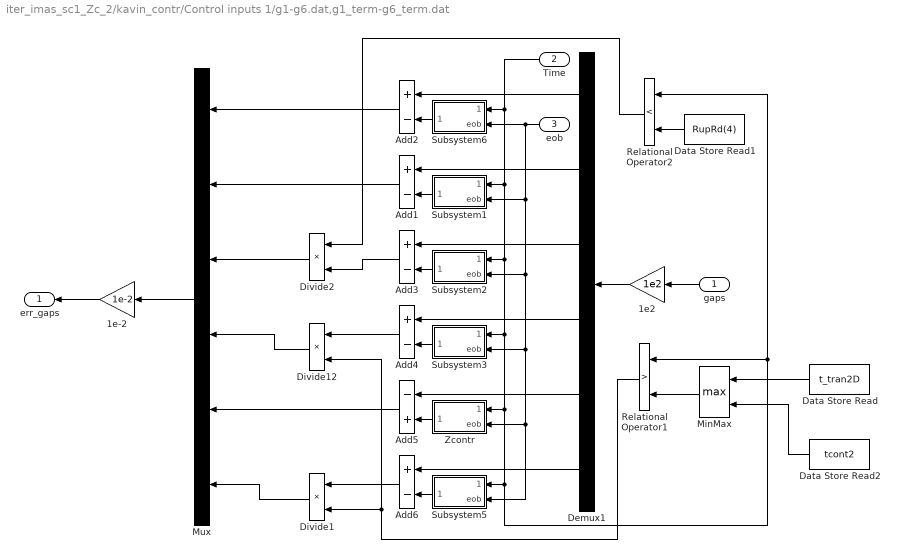
== system iter_imas_sc1_Zc_2/kavin_contr/Control inputs 1/g1-g6.dat,g1_term-g6_term.dat ==
  gaps : Inport
  Time : Inport  Port=2
  eob : Inport  Port=3
  1e-2 : Gain  Gain=1e-2
  1e2 : Gain  Gain=1e2
  Add{1..4,6} (5 alike) : Sum  Inputs=+-
  Add5 : Sum  Inputs=-+
  Data Store Read : DataStoreRead  DataStoreName=t_tran2D  DataStoreElements=t_tran2D
  Data Store Read1 : DataStoreRead  DataStoreName=RupRd  DataStoreElements=RupRd(4)
  Data Store Read2 : DataStoreRead  DataStoreName=tcont2  DataStoreElements=tcont2
  Demux1 : Demux  Outputs=6
  Divide1 : Product  Inputs=**
  Divide12 : Product  Inputs=**
  Divide2 : Product  Inputs=**
  MinMax : MinMax  Function=max  Inputs=2
  Mux : Mux  Inputs=6
  Relational Operator1 : RelationalOperator  Operator=>  OutDataTypeStr=float('double')
  Relational Operator2 : RelationalOperator  Operator=<  OutDataTypeStr=float('double')
  Subsystem1 : Subsystem
  Subsystem2 : Subsystem
  Subsystem3 : Subsystem
  Subsystem5 : Subsystem
  Subsystem6 : Subsystem
  Zcontr : Subsystem
  err_gaps : Outport
  wires:
  gaps/1 -> 1e2/1
  Time/1 -> Relational Operator2/1, Relational Operator1/1, Subsystem5/1(Time), Zcontr/1(Time), Subsystem3/1(Time), Subsystem2/1(Time), Subsystem1/1(Time), Subsystem6/1(Time)
  Demux1/1 -> Add2/1
  Demux1/2 -> Add1/1
  Subsystem1/1(Out1) -> Add1/2
  Subsystem2/1(Out1) -> Add3/2
  Demux1/3 -> Add3/1
  Demux1/4 -> Add4/1
  Subsystem3/1(Out1) -> Add4/2
  Demux1/5 -> Add5/1
  Zcontr/1(Out1) -> Add5/2
  Demux1/6 -> Add6/1
  1e2/1 -> Demux1/1
  1e-2/1 -> err_gaps/1
  Subsystem6/1(Out1) -> Add2/2
  eob/1 -> Subsystem1/2(eob), Subsystem2/2(eob), Subsystem3/2(eob), Zcontr/2(eob), Subsystem5/2(eob), Subsystem6/2(eob)
  Subsystem5/1(Out1) -> Add6/2
  Mux/1 -> 1e-2/1
  Add2/1 -> Mux/1
  Add1/1 -> Mux/2
  Add5/1 -> Mux/5
  Add4/1 -> Divide12/1
  Divide12/1 -> Mux/4
  Relational Operator1/1 -> Divide1/2, Divide12/2
  Add6/1 -> Divide1/1
  Divide1/1 -> Mux/6
  Data Store Read1/1 -> Relational Operator2/2
  Divide2/1 -> Mux/3
  Add3/1 -> Divide2/2
  Relational Operator2/1 -> Divide2/1
  MinMax/1 -> Relational Operator1/2
  Data Store Read/1 -> MinMax/1
  Data Store Read2/1 -> MinMax/2

== system iter_imas_sc1_Zc_2/kavin_contr/Control inputs 1/g4 ==
  gaps3-6 : Inport
  Constant1 : Constant  VectorParams1D=off
  Constant2 : Constant  VectorParams1D=off
  Constant4 : Constant  VectorParams1D=off
  Data Store Read1 : DataStoreRead  DataStoreName=k_g4  DataStoreElements=k_g4
  Divide : Product  Inputs=**
  Mux : Mux
  glim : Outport
  wires:
  gaps3-6/1 -> Divide/1
  Divide/1 -> glim/1
  Mux/1 -> Divide/2
  Constant4/1 -> Mux/1
  Constant1/1 -> Mux/3
  Constant2/1 -> Mux/4
  Data Store Read1/1 -> Mux/2

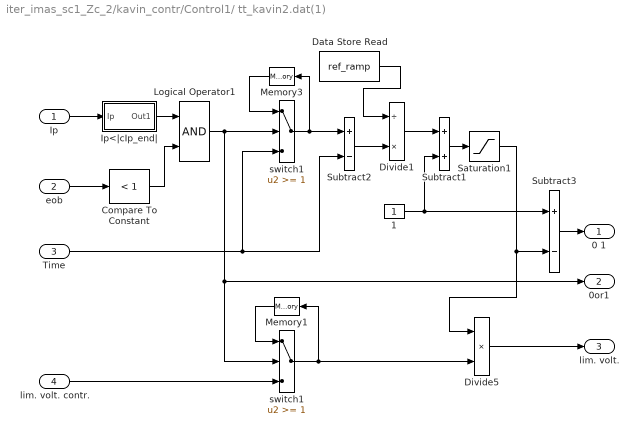
== system iter_imas_sc1_Zc_2/kavin_contr/Control1/ tt_kavin2.dat(1) ==
  Ip : Inport
  eob : Inport  Port=2
  Time : Inport  Port=3
  lim. volt. contr. : Inport  Port=4
  1 : Constant
  Compare To Constant : simulink/Logic and Bit Operations/Compare To Constant  relop=<  const=1  OutDataTypeStr=boolean  ZeroCross=off
  Data Store Read : DataStoreRead  DataStoreName=ref_ramp  DataStoreElements=ref_ramp
  Divide1 : Product  Inputs=/*
  Divide5 : Product  Inputs=**
  Ip<|cIp_end| : Subsystem
  Logical Operator1 : Logic  AllPortsSameDT=off  OutDataTypeStr=float('double')
  Memory1 : Memory
  Memory3 : Memory
  Saturation1 : Saturate  UpperLimit=1  LowerLimit=0
  Subtract1 : Sum
  Subtract2 : Sum  Inputs=+-
  Subtract3 : Sum  Inputs=+-
  switch1 : Switch  Threshold=1
  "switch1 " : Switch  Threshold=1
  0 1 : Outport
  0or1 : Outport  Port=2
  "lim. volt. " : Outport  Port=3
  wires:
  "switch1 "/1 -> Memory3/1, Subtract2/1
  Memory3/1 -> "switch1 "/1
  Subtract2/1 -> Divide1/2
  eob/1 -> Compare To Constant/1
  Ip/1 -> Ip<|cIp_end|/1(Ip)
  Ip<|cIp_end|/1(Out1) -> Logical Operator1/1
  Compare To Constant/1 -> Logical Operator1/2
  Logical Operator1/1 -> "switch1 "/2, switch1/2, 0or1/1
  Divide1/1 -> Subtract1/1
  Subtract1/1 -> Saturation1/1
  Saturation1/1 -> Divide5/1, Subtract3/2
  1/1 -> Subtract1/2, Subtract3/1
  Subtract3/1 -> 0 1/1
  Time/1 -> Subtract2/2, "switch1 "/3
  lim. volt. contr./1 -> switch1/3
  switch1/1 -> Memory1/1, Divide5/2
  Memory1/1 -> switch1/1
  Divide5/1 -> "lim. volt. "/1
  Data Store Read/1 -> Divide1/1

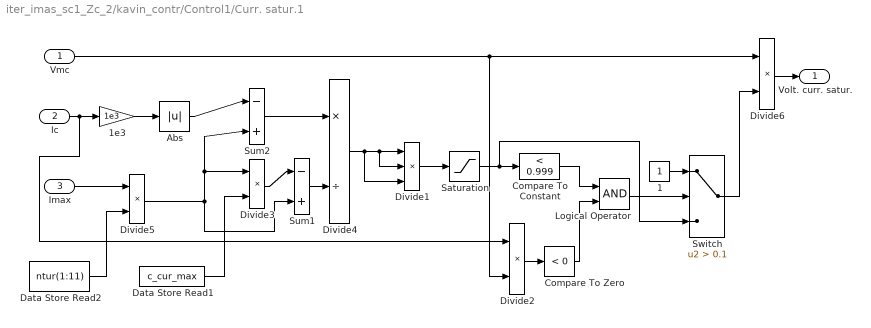
== system iter_imas_sc1_Zc_2/kavin_contr/Control1/Curr. satur.1 ==
  Vmc : Inport
  Ic : Inport  Port=2
  Imax : Inport  Port=3
  1 : Constant
  1e3 : Gain  Gain=1e3
  Abs : Abs
  Compare To Constant : simulink/Logic and Bit Operations/Compare To Constant  relop=<  const=0.999  OutDataTypeStr=uint8  ZeroCross=off
  Compare To Zero : simulink/Logic and Bit Operations/Compare To Zero  relop=<  OutDataTypeStr=uint8  ZeroCross=off
  Data Store Read1 : DataStoreRead  DataStoreName=c_cur_max  DataStoreElements=c_cur_max
  Data Store Read2 : DataStoreRead  DataStoreName=ntur  DataStoreElements=ntur(1:11)
  Divide1 : Product  Inputs=***
  Divide{2..3,5..6} (4 alike) : Product  Inputs=**
  Divide4 : Product  Inputs=*/
  Logical Operator : Logic  AllPortsSameDT=off  OutDataTypeStr=boolean
  Saturation : Saturate  UpperLimit=1  LowerLimit=-1
  Sum1 : Sum  Inputs=|-+
  Sum2 : Sum  Inputs=|-+
  Switch : Switch  Criteria=u2 > Threshold  Threshold=0.1
  Volt. curr. satur. : Outport
  wires:
  Ic/1 -> 1e3/1, Divide2/1
  1e3/1 -> Abs/1
  Imax/1 -> Divide5/1
  Abs/1 -> Sum2/1
  Divide5/1 -> Divide3/1, Sum2/2, Sum1/2
  Divide3/1 -> Sum1/1
  Sum2/1 -> Divide4/1
  Sum1/1 -> Divide4/2
  Divide4/1 -> Divide1/3, Divide1/1, Divide1/2
  Divide1/1 -> Saturation/1
  Vmc/1 -> Divide6/1, Divide2/2
  Divide6/1 -> Volt. curr. satur./1
  Saturation/1 -> Switch/3, Compare To Constant/1
  Divide2/1 -> Compare To Zero/1
  Compare To Constant/1 -> Logical Operator/1
  Compare To Zero/1 -> Logical Operator/2
  Switch/1 -> Divide6/2
  Data Store Read1/1 -> Divide3/2
  Data Store Read2/1 -> Divide5/2
  Logical Operator/1 -> Switch/2
  1/1 -> Switch/1

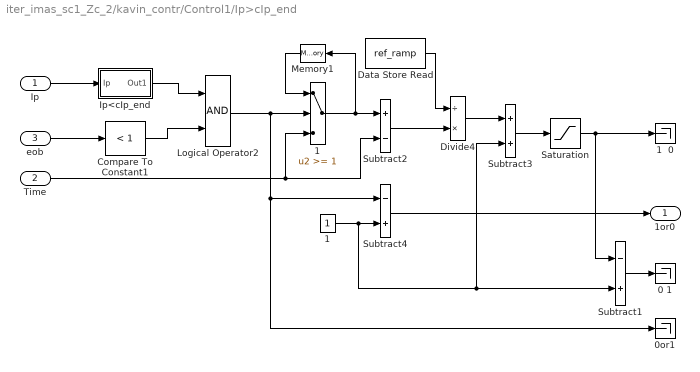
== system iter_imas_sc1_Zc_2/kavin_contr/Control1/Ip>cIp_end ==
  Ip : Inport
  Time : Inport  Port=2
  eob : Inport  Port=3
  0 1 : Terminator
  0or1 : Terminator
  1 : Constant
  "1 " : Switch  Threshold=1
  1  0 : Terminator
  Compare To Constant1 : simulink/Logic and Bit Operations/Compare To Constant  relop=<  const=1  OutDataTypeStr=boolean  ZeroCross=off
  Data Store Read : DataStoreRead  DataStoreName=ref_ramp  DataStoreElements=ref_ramp
  Divide4 : Product  Inputs=/*
  Ip<cIp_end : Subsystem
  Logical Operator2 : Logic  AllPortsSameDT=off  OutDataTypeStr=float('double')
  Memory1 : Memory
  Saturation : Saturate  UpperLimit=1  LowerLimit=0
  Subtract1 : Sum  Inputs=-+
  Subtract2 : Sum  Inputs=+-
  Subtract3 : Sum
  Subtract4 : Sum  Inputs=-+
  1or0 : Outport
  wires:
  Logical Operator2/1 -> "1 "/2, 0or1/1, Subtract4/1
  Time/1 -> Subtract2/2, "1 "/3
  "1 "/1 -> Memory1/1, Subtract2/1
  Memory1/1 -> "1 "/1
  Subtract2/1 -> Divide4/2
  Divide4/1 -> Subtract3/1
  1/1 -> Subtract3/2, Subtract1/2, Subtract4/2
  Subtract3/1 -> Saturation/1
  Subtract1/1 -> 0 1/1
  Compare To Constant1/1 -> Logical Operator2/2
  Ip<cIp_end/1(Out1) -> Logical Operator2/1
  Ip/1 -> Ip<cIp_end/1(Ip)
  Saturation/1 -> Subtract1/1, 1  0/1
  Data Store Read/1 -> Divide4/1
  eob/1 -> Compare To Constant1/1
  Subtract4/1 -> 1or0/1

== system iter_imas_sc1_Zc_2/kavin_contr/Control1/Lim. contr.1 ==
  err lim : Inport
  Time : Inport  Port=2
  atpl2 : Inport  Port=3
  1e6 : Gain  Gain=1e6
  Curr. contr. : DiscreteStateSpace  A=Acd2  B=Bcd2  C=Ccd2  D=Dcd2  SampleTime=SimStep
  Data Store Read2 : DataStoreRead  DataStoreName=ntur  DataStoreElements=ntur(1:11)
  "Divide " : Product  Inputs=***
  Divide1 : Product  Inputs=*/
  Divide2 : Product  Inputs=*/
  Lim. contr. : DiscreteStateSpace  A=A_lim  B=B_lim  C=C_lim  D=D_lim  SampleTime=SimStep
  err Ipf : Selector  InputPortWidth=20  Indices=[9:19]
  gain_cont2 : Subsystem
  t_cont2 : Subsystem
  t_cont2_2 : Subsystem
  lim. volt. : Outport
  wires:
  err lim/1 -> t_cont2/1(errlim), err Ipf/1
  Time/1 -> t_cont2_2/2(Time), t_cont2/2(Time), gain_cont2/1(Time)
  Divide1/1 -> 1e6/1
  Curr. contr./1 -> Divide2/1
  t_cont2/1(Out1) -> Lim. contr./1
  err Ipf/1 -> Divide1/1
  Data Store Read2/1 -> Divide1/2, Divide2/2
  "Divide "/1 -> t_cont2_2/1(lim. contr.)
  Divide2/1 -> t_cont2_2/3(Curr. cont.)
  t_cont2_2/1(Out1) -> lim. volt./1
  1e6/1 -> Curr. contr./1
  gain_cont2/1(Out1) -> "Divide "/3
  Lim. contr./1 -> "Divide "/2
  atpl2/1 -> "Divide "/1

== system iter_imas_sc1_Zc_2/kavin_contr/Control1/Subsystem7 ==
  Ip : Inport
  Udiv : Inport  Port=2
  eob : Inport  Port=3
  0.1 : Switch  Threshold=0.1
  Abs : Abs
  Compare To Constant1 : simulink/Logic and Bit Operations/Compare To Constant  relop=<  const=1  OutDataTypeStr=boolean  ZeroCross=off
  Data Store Read : DataStoreRead  DataStoreName=Ip_rd  DataStoreElements=Ip_rd
  Data Store Read1 : DataStoreRead  DataStoreName=RupRd  DataStoreElements=RupRd(3)
  Logical Operator1 : Logic  Inputs=3  AllPortsSameDT=off  OutDataTypeStr=float('double')
  Memory : Memory
  Relational Operator : RelationalOperator  Operator=>  OutDataTypeStr=boolean
  Relational Operator1 : RelationalOperator  Operator=<  OutDataTypeStr=boolean
  "Udiv " : Outport
  wires:
  Ip/1 -> Relational Operator1/1, Relational Operator/1
  Relational Operator1/1 -> Logical Operator1/1
  Compare To Constant1/1 -> Logical Operator1/2
  Udiv/1 -> 0.1/3
  Memory/1 -> 0.1/1
  Logical Operator1/1 -> 0.1/2
  0.1/1 -> Memory/1, "Udiv "/1
  Data Store Read1/1 -> Abs/1
  Abs/1 -> Relational Operator/2
  Relational Operator/1 -> Logical Operator1/3
  Data Store Read/1 -> Relational Operator1/2
  eob/1 -> Compare To Constant1/1

== system iter_imas_sc1_Zc_2/kavin_contr/Control1/Subsystem8 ==
  VSrd : Inport
  VSeob : Inport  Port=2
  eob : Inport  Port=3
  Ipl : Inport  Port=4
  1 : Switch  Threshold=1
  Abs : Abs
  Compare To Constant1 : simulink/Logic and Bit Operations/Compare To Constant  relop=<  const=1  OutDataTypeStr=boolean  ZeroCross=off
  Data Store Read : DataStoreRead  DataStoreName=RupRd  DataStoreElements=RupRd(3)
  Data Store Read1 : DataStoreRead  DataStoreName=Ip_rd  DataStoreElements=Ip_rd
  Logical Operator1 : Logic  Inputs=3  AllPortsSameDT=off  OutDataTypeStr=float('double')
  Relational Operator1 : RelationalOperator  Operator=>  OutDataTypeStr=float('double')
  Relational Operator2 : RelationalOperator  Operator=<  OutDataTypeStr=float('double')
  Out1 : Outport
  wires:
  1/1 -> Out1/1
  VSeob/1 -> 1/3
  VSrd/1 -> 1/1
  Data Store Read/1 -> Abs/1
  Abs/1 -> Relational Operator1/2
  Ipl/1 -> Relational Operator1/1, Relational Operator2/1
  Logical Operator1/1 -> 1/2
  Relational Operator1/1 -> Logical Operator1/2
  Relational Operator2/1 -> Logical Operator1/1
  eob/1 -> Compare To Constant1/1
  Compare To Constant1/1 -> Logical Operator1/3
  Data Store Read1/1 -> Relational Operator2/2

== system iter_imas_sc1_Zc_2/kavin_contr/Control1/VS VShl contr. ==
  err VS : Inport
  eob : Inport  Port=2
  Compare To Constant1 : simulink/Logic and Bit Operations/Compare To Constant  relop=<  const=1  OutDataTypeStr=boolean  ZeroCross=off
  Divide4 : Product  Inputs=**
  VS. contr : DiscreteStateSpace  A=A_vs  B=B_vs  C=C_vs  D=D_vs  SampleTime=SimStep
  VS. contr hl : DiscreteStateSpace  A=A_vs_hl  B=B_vs_hl  C=C_vs_hl  D=D_vs_hl  SampleTime=SimStep
  c_eob : Switch  Threshold=1
  Out1 : Outport
  wires:
  eob/1 -> c_eob/2, Compare To Constant1/1
  VS. contr/1 -> c_eob/1
  VS. contr hl/1 -> c_eob/3
  err VS/1 -> VS. contr/1, Divide4/2
  c_eob/1 -> Out1/1
  Divide4/1 -> VS. contr hl/1
  Compare To Constant1/1 -> Divide4/1

== system iter_imas_sc1_Zc_2/kavin_contr/Control1/VS gain 1 ==
  Ipl : Inport
  1 : Constant  Value=0
  1/15 : Gain  Gain=1/15
  Data Store Read : DataStoreRead  DataStoreName=c_a_tpl1  DataStoreElements=c_a_tpl1
  Data Store Read1 : DataStoreRead  DataStoreName=Ip_div  DataStoreElements=Ip_div
  Data Store Read2 : DataStoreRead  DataStoreName=max_VS_lim  DataStoreElements=max_VS_lim
  Div : Product  Inputs=**
  Lim. Div. tr. : Switch  Threshold=1
  Relational Operator2 : RelationalOperator  Operator=>  OutDataTypeStr=float('double')
  Sat. Div : Saturate  UpperLimit=1  LowerLimit=0
  Saturation Dynamic : simulink/Discontinuities/Saturation Dynamic  OutMin=[]  OutMax=[]  OutDataTypeStr=Inherit: Same as second input  OutDataType=fixdt(1, 16)  OutScaling=2^-10  DoSatur=off
  VS gain : Outport
  wires:
  Lim. Div. tr./1 -> VS gain/1
  Saturation Dynamic/1 -> Lim. Div. tr./3
  Sat. Div/1 -> Lim. Div. tr./1
  Data Store Read/1 -> 1/15/1
  1/15/1 -> Div/2
  Div/1 -> Saturation Dynamic/2, Sat. Div/1
  Ipl/1 -> Relational Operator2/1, Div/1
  Data Store Read1/1 -> Relational Operator2/2
  Relational Operator2/1 -> Lim. Div. tr./2
  1/1 -> Saturation Dynamic/3
  Data Store Read2/1 -> Saturation Dynamic/1

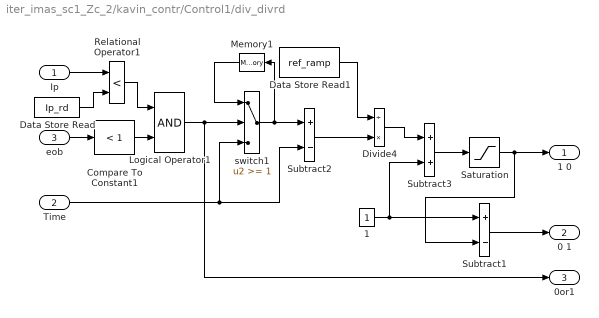
== system iter_imas_sc1_Zc_2/kavin_contr/Control1/div_divrd ==
  Ip : Inport
  Time : Inport  Port=2
  eob : Inport  Port=3
  1 : Constant
  Compare To Constant1 : simulink/Logic and Bit Operations/Compare To Constant  relop=<  const=1  OutDataTypeStr=boolean  ZeroCross=off
  Data Store Read : DataStoreRead  DataStoreName=Ip_rd  DataStoreElements=Ip_rd
  Data Store Read1 : DataStoreRead  DataStoreName=ref_ramp  DataStoreElements=ref_ramp
  Divide4 : Product  Inputs=/*
  Logical Operator1 : Logic  AllPortsSameDT=off  OutDataTypeStr=float('double')
  Memory1 : Memory
  Relational Operator1 : RelationalOperator  Operator=<  OutDataTypeStr=boolean
  Saturation : Saturate  UpperLimit=1  LowerLimit=0
  Subtract1 : Sum  Inputs=+-
  Subtract2 : Sum  Inputs=+-
  Subtract3 : Sum
  switch1 : Switch  Threshold=1
  1 0 : Outport
  0 1 : Outport  Port=2
  0or1 : Outport  Port=3
  wires:
  Time/1 -> switch1/3, Subtract2/2
  Logical Operator1/1 -> switch1/2, 0or1/1
  switch1/1 -> Subtract2/1, Memory1/1
  Memory1/1 -> switch1/1
  Subtract2/1 -> Divide4/2
  Divide4/1 -> Subtract3/1
  Subtract3/1 -> Saturation/1
  Saturation/1 -> Subtract1/2, 1 0/1
  1/1 -> Subtract1/1, Subtract3/2
  Subtract1/1 -> 0 1/1
  Data Store Read1/1 -> Divide4/1
  eob/1 -> Compare To Constant1/1
  Compare To Constant1/1 -> Logical Operator1/2
  Relational Operator1/1 -> Logical Operator1/1
  Data Store Read/1 -> Relational Operator1/2
  Ip/1 -> Relational Operator1/1

== system iter_imas_sc1_Zc_2/kavin_contr/Control1/dzdt noise1 ==
  VS3 inputs : Inport
  Time : Inport  Port=2
  Demux : Demux  Outputs=[1 1]
  Mux : Mux  Inputs=2
  Subsystem : Subsystem
  Sum2 : Sum  Inputs=|++
  Uniform Random Number : UniformRandomNumber  SampleTime=SimStep
  Out1 : Outport
  wires:
  VS3 inputs/1 -> Demux/1
  Demux/1 -> Sum2/2
  Sum2/1 -> Mux/1
  Demux/2 -> Mux/2
  Mux/1 -> Out1/1
  Uniform Random Number/1 -> Subsystem/1(Noise)
  Time/1 -> Subsystem/2(Time)
  Subsystem/1(Out1) -> Sum2/1

== system iter_imas_sc1_Zc_2/kavin_contr/Control1/scr_data.dat ==
  eob : Inport
  Ipl : Inport  Port=2
  1 : Constant
  2 : Constant
  Data Store Read2 : DataStoreRead  DataStoreName=y0  DataStoreElements=y0
  Data Store Read3 : DataStoreRead  DataStoreName=c1_y0  DataStoreElements=c1_y0
  Data Store Read4 : DataStoreRead  DataStoreName=c2_y0  DataStoreElements=c2_y0
  Divide1 : Product  Inputs=/*
  Divide2 : Product  Inputs=**
  Divide6 : Product  Inputs=**
  Memory1 : Memory
  Saturation Dynamic : simulink/Discontinuities/Saturation Dynamic  OutMin=[]  OutMax=[]  OutDataTypeStr=Inherit: Same as second input  OutDataType=fixdt(1, 16)  OutScaling=2^-10  DoSatur=off
  Sum : Sum  Inputs=|+-
  Sum1 : Sum  Inputs=|++
  Sum2 : Sum  Inputs=+-
  Sum3 : Sum  Inputs=+-
  c_eob : Switch  Threshold=1
  gain rd : Outport
  wires:
  Data Store Read3/1 -> Sum2/2, Sum/2
  Data Store Read2/1 -> Sum3/2, Sum1/2, Saturation Dynamic/3
  Sum1/1 -> Saturation Dynamic/2
  Divide2/1 -> Sum1/1
  Sum/1 -> Divide2/1
  Saturation Dynamic/1 -> gain rd/1
  Divide6/1 -> Sum/1
  c_eob/1 -> Divide6/1, Memory1/1
  eob/1 -> c_eob/2, Divide6/2
  Memory1/1 -> c_eob/3
  Ipl/1 -> c_eob/1
  1/1 -> Saturation Dynamic/1
  Data Store Read4/1 -> Sum2/1
  2/1 -> Sum3/1
  Sum3/1 -> Divide1/2
  Sum2/1 -> Divide1/1
  Divide1/1 -> Divide2/2

== system iter_imas_sc1_Zc_2/kavin_contr/Control1/t_tran2D ==
  Noise,VS3 : Inport
  Time : Inport  Port=2
  Data Store Read : DataStoreRead  DataStoreName=t_tran2D  DataStoreElements=t_tran2D
  Data Store Read2 : DataStoreRead  DataStoreName=tcont2  DataStoreElements=tcont2
  Divide12 : Product  Inputs=**
  MinMax : MinMax  Function=max  Inputs=2
  Relational Operator1 : RelationalOperator  Operator=>  OutDataTypeStr=float('double')
  Out1 : Outport
  wires:
  Noise,VS3/1 -> Divide12/1
  Time/1 -> Relational Operator1/1
  Relational Operator1/1 -> Divide12/2
  Divide12/1 -> Out1/1
  MinMax/1 -> Relational Operator1/2
  Data Store Read/1 -> MinMax/1
  Data Store Read2/1 -> MinMax/2
